simulink model "FSK"  (R2023b)
settings: Solver=VariableStepAuto  StartTime=0.0  StopTime=10.0  RelTol=1e-3
settings Model: Creator=satyamagrawal  LastModifiedBy=satyamagrawal

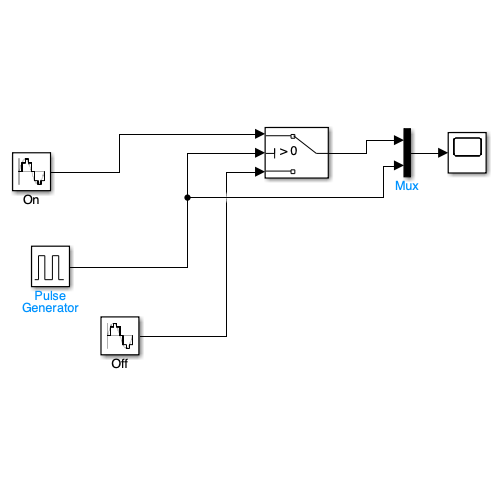
[thumbnail: Simulink's stored preview of the top-level diagram]
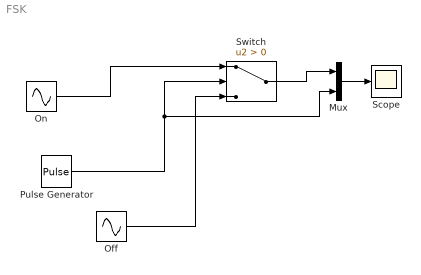
== system FSK ==
  Mux : Mux  Inputs=2
  Off : Sin  Frequency=20  SampleTime=0.0001
  On : Sin  Frequency=40  SampleTime=0.0001
  Pulse Generator : DiscretePulseGenerator  PulseType=Time based  PulseWidth=50
  Scope : Scope
  Switch : Switch  Criteria=u2 > Threshold  SaturateOnIntegerOverflow=off  InputSameDT=off
  wires:
  Pulse Generator/1 -> Mux/2, Switch/2
  On/1 -> Switch/1
  Off/1 -> Switch/3
  Switch/1 -> Mux/1
  Mux/1 -> Scope/1
